simulink model "full_system_nios_id3"  (R2021b)
settings: Solver=FixedStepDiscrete  StartTime=0.0  StopTime=250000  RelTol=1e-3
model workspace (MAT data in the model file):
  out_size = 0
undefined symbols (not defined in the file): betas, bias, DiscIntNeverNeededParam, mus, scale, sigmas
libraries: hdlsllib x2
settings Model: DataTypeOverride=Off  SimulationMode=accelerator  Creator=local_adm  LastModifiedBy=local_adm
settings SolverCC: AlgebraicLoopSolver=TrustRegion
settings DataIOCC: LimitDataPoints=on  SaveOutput=off  SaveTime=off
settings OptimizationCC: BlockReduction=off  ConditionallyExecuteInputs=off  DefaultParameterBehavior=Inlined  LifeSpan=inf
settings DebuggingCC: AlgebraicLoopMsg=error  SingleTaskRateTransMsg=error  ParameterPrecisionLossMsg=none  AllowSymbolicDim=off  StrictBusMsg=ErrorOnBusTreatedAsVector  SFUnexpectedBacktrackingDiag=warning  SFNoUnconditionalDefaultTransitionDiag=warning  SFExecutionAtInitializationDiag=none  SFMachineParentedDataDiag=warning  ArithmeticOperatorsInVariantConditions=warning
settings HardwareCC: ProdBitPerPointer=32  ProdBitPerSizeT=32  ProdBitPerPtrDiffT=32  ProdLargestAtomicFloat=None  ProdIntDivRoundTo=Undefined  ProdEndianess=Unspecified  ProdWordSize=32  ProdHWDeviceType=ASIC/FPGA->ASIC/FPGA  ProdEqTarget=off
settings SFSimCC: SimUseLocalCustomCode=off  CustomCodeUndefinedFunction=UseInterfaceOnly
settings RTWCC: RTWUseLocalCustomCode=off
settings CodeAppCC: StateflowObjectComments=on
settings GRTTargetCC: TargetLangStandard=C89/C90 (ANSI)
settings ConfigComp: CovScope=ReferencedModels  CovMetricSettings=dw  CovSaveCumulativeToWorkspaceVar=on  CovSaveSingleToWorkspaceVar=on  CovExternalEMLEnable=off  CovSFcnEnable=off

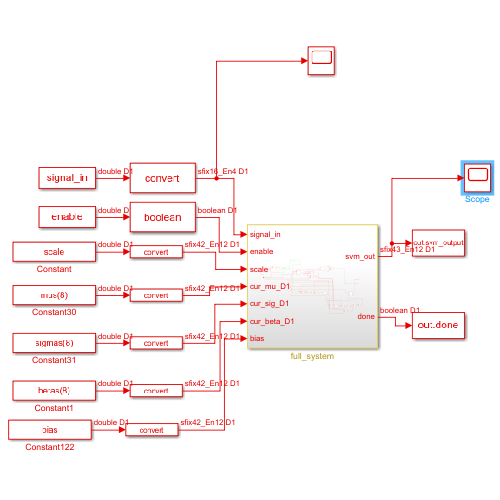
[thumbnail: Simulink's stored preview of the top-level diagram]
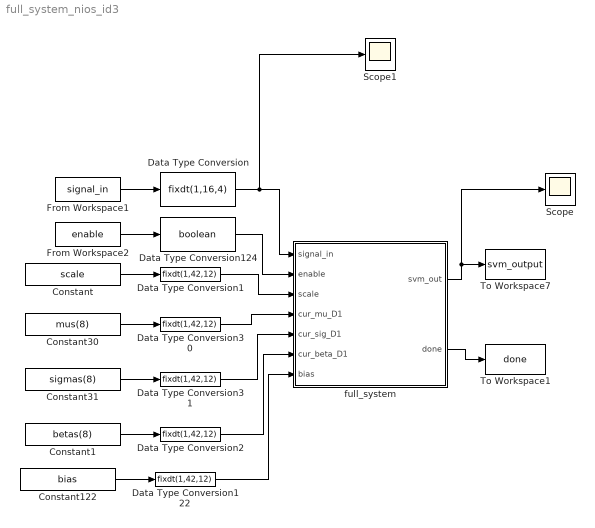
== system full_system_nios_id3 ==
  Constant : Constant  Value=scale  VectorParams1D=off  SampleTime=-1
  Constant1 : Constant  Value=betas(8)  VectorParams1D=off  SampleTime=-1
  Constant122 : Constant  Value=bias  VectorParams1D=off  SampleTime=-1
  Constant30 : Constant  Value=mus(8)  VectorParams1D=off  SampleTime=-1
  Constant31 : Constant  Value=sigmas(8)  VectorParams1D=off  SampleTime=-1
  Data Type Conversion : DataTypeConversion  OutMax=2  OutDataTypeStr=fixdt(1,16,4)
  Data Type Conversion{1..2,30..31,122} (5 alike) : DataTypeConversion  OutMax=2  OutDataTypeStr=fixdt(1,42,12)
  Data Type Conversion124 : DataTypeConversion  OutMax=1  OutDataTypeStr=boolean
  From Workspace1 : FromWorkspace  VariableName=signal_in  SampleTime=1  OutputAfterFinalValue=Setting to zero
  From Workspace2 : FromWorkspace  VariableName=enable  SampleTime=1  OutputAfterFinalValue=Setting to zero
  Scope : Scope
  Scope1 : Scope
  To Workspace1 : ToWorkspace  VariableName=done  SampleTime=-1
  To Workspace7 : ToWorkspace  VariableName=svm_output  SampleTime=-1
  full_system : Subsystem
  wires:
  full_system/2(done) -> To Workspace1/1
  From Workspace2/1 -> Data Type Conversion124/1
  Data Type Conversion30/1 -> full_system/4(cur_mu_D1)
  Data Type Conversion122/1 -> full_system/7(bias)
  Data Type Conversion31/1 -> full_system/5(cur_sig_D1)
  Data Type Conversion1/1 -> full_system/3(scale)
  Data Type Conversion124/1 -> full_system/2(enable)
  Data Type Conversion/1 -> Scope1/1, full_system/1(signal_in)
  Constant122/1 -> Data Type Conversion122/1
  full_system/1(svm_out) -> Scope/1, To Workspace7/1
  Constant30/1 -> Data Type Conversion30/1
  Constant31/1 -> Data Type Conversion31/1
  Constant/1 -> Data Type Conversion1/1
  From Workspace1/1 -> Data Type Conversion/1
  Constant1/1 -> Data Type Conversion2/1
  Data Type Conversion2/1 -> full_system/6(cur_beta_D1)

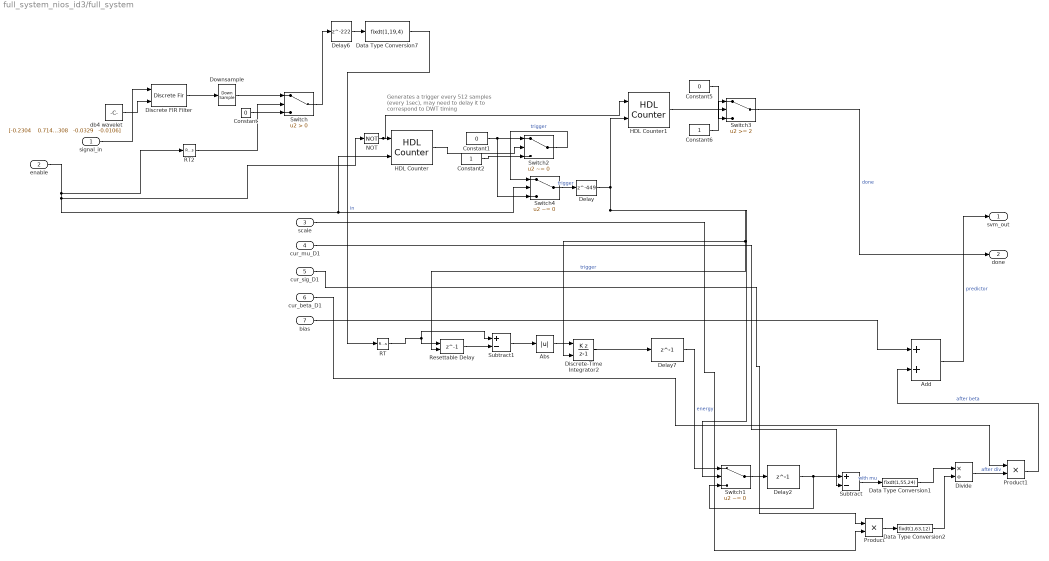
== system full_system_nios_id3/full_system ==
  note: Generates a trigger every 512 samples (every 1sec), may need to delay it to correspond to DWT timing
  signal_in : Inport
  enable : Inport  Port=2
  scale : Inport  Port=3
  cur_mu_D1 : Inport  Port=4
  cur_sig_D1 : Inport  Port=5
  cur_beta_D1 : Inport  Port=6
  bias : Inport  Port=7
  Abs : Abs
  Add : Sum
  Constant : Constant  Value=0  OutDataTypeStr=Inherit: Inherit via back propagation  SampleTime=-1
  Constant1 : Constant  Value=0  VectorParams1D=off  OutDataTypeStr=boolean  SampleTime=-1
  Constant2 : Constant  VectorParams1D=off  OutDataTypeStr=boolean  SampleTime=-1
  Constant5 : Constant  Value=0  VectorParams1D=off  OutDataTypeStr=boolean  SampleTime=-1
  Constant6 : Constant  VectorParams1D=off  OutDataTypeStr=boolean  SampleTime=-1
  Data Type Conversion1 : DataTypeConversion  OutMax=2  OutDataTypeStr=fixdt(1,55,24)
  Data Type Conversion2 : DataTypeConversion  OutMax=2  OutDataTypeStr=fixdt(1,63,12)
  Data Type Conversion7 : DataTypeConversion  OutDataTypeStr=fixdt(1,19,4)
  Delay : Delay  DelayLength=449  InitialCondition=0  UseCircularBuffer=on
  Delay2 : Delay  DelayLength=1  InitialCondition=0  UseCircularBuffer=on
  Delay6 : Delay  DelayLength=222
  Delay7 : Delay  DelayLength=1  InitialCondition=0  UseCircularBuffer=on
  Discrete FIR Filter : DiscreteFir  CoefSource=Input port
      settings: InputPortMap=u0,u1
  Discrete-Time Integrator2 : DiscreteIntegrator  IntegratorMethod=Accumulation: Backward Euler  ExternalReset=rising  SampleTime=-1  ICPrevOutput=DiscIntNeverNeededParam  ICPrevScaledInput=DiscIntNeverNeededParam
  Divide : Product  Inputs=*/  OutDataTypeStr=fixdt(1,42,12)  RndMeth=Zero  SaturateOnIntegerOverflow=on
  Downsample : DownSample  phase=1  RateOptions=Allow multirate processing
  HDL Counter : hdlsllib/Sources/HDL Counter  CountType=Count limited  CountInit=0  CountStep=1  CountMax=511  CountFromType=Initial value  CountFrom=0  CountResetPort=on  CountLoadPort=off  CountEnbPort=on  CountDirPort=off  CountHitOutputPort=off  CountDataType=Unsigned  CountWordLen=9  CountFracLen=0  CountSampTime=1
  HDL Counter1 : hdlsllib/Sources/HDL Counter  CountType=Count limited  CountInit=0  CountStep=1  CountMax=2  CountFromType=Initial value  CountFrom=0  CountResetPort=on  CountLoadPort=off  CountEnbPort=on  CountDirPort=off  CountHitOutputPort=off  CountDataType=Unsigned  CountWordLen=4  CountFracLen=0  CountSampTime=1
  NOT : Logic  Operator=NOT  IconShape=distinctive  AllPortsSameDT=off  OutDataTypeStr=boolean
  Product : Product
  Product1 : Product  OutDataTypeStr=fixdt(1,32,12)
  RT : RateTransition  OutPortSampleTime=1
  RT2 : RateTransition  OutPortSampleTime=2
  Resettable Delay : Delay  DelayLength=1  ExternalReset=Level
      settings: InputPortMap=u0,r5
  Subtract : Sum  Inputs=+-
  Subtract1 : Sum  Inputs=+-
  Switch : Switch  Criteria=u2 > Threshold
  Switch1 : Switch  Criteria=u2 ~= 0
  Switch2 : Switch  Criteria=u2 ~= 0
  Switch3 : Switch  Threshold=2
  Switch4 : Switch  Criteria=u2 ~= 0
  db4 wavelet : Constant  Value="[-0.2304    0.7148   -0.6309   -0.0280    0.1870    0.0308   -0.0329   -0.0106]"  OutDataTypeStr=Inherit: Inherit via back propagation  SampleTime=-1
  svm_out : Outport
  done : Outport  Port=2
  wires:
  Switch/1 -> Delay6/1
  Delay6/1 -> Data Type Conversion7/1
  RT2/1 -> Switch/2
  Downsample/1 -> Switch/1
  Discrete FIR Filter/1 -> Downsample/1
  Constant/1 -> Switch/3
  signal_in/1 -> Discrete FIR Filter/1
  db4 wavelet/1 -> Discrete FIR Filter/2
  Resettable Delay/1 -> Subtract1/2
  Subtract1/1 -> Abs/1
  Abs/1 -> Discrete-Time Integrator2/1
  Discrete-Time Integrator2/1 -> Delay7/1
  RT/1 -> Resettable Delay/1, Subtract1/1
  Data Type Conversion7/1 -> RT/1  "in"
  Switch3/1 -> done/1  "done"
  HDL Counter1/1 -> Switch3/2
  Constant6/1 -> Switch3/1
  Constant5/1 -> Switch3/3
  NOT/1 -> HDL Counter1/1, HDL Counter/1
  Switch4/1 -> Delay/1  "trigger"
  Switch2/1 -> Switch4/1  "trigger"
  enable/1 -> Switch4/2, HDL Counter/2, NOT/1, RT2/1
  Add/1 -> svm_out/1  "predictor"
  bias/1 -> Add/1
  Delay/1 -> Switch1/2, Resettable Delay/2, Discrete-Time Integrator2/2, HDL Counter1/2  "trigger"
  Constant1/1 -> Switch4/3, Switch2/1
  Constant2/1 -> Switch2/3
  HDL Counter/1 -> Switch2/2
  Divide/1 -> Product1/2  "after div"
  Product1/1 -> Add/2  "after beta"
  Data Type Conversion2/1 -> Divide/2
  cur_beta_D1/1 -> Product1/1
  Switch1/1 -> Delay2/1
  scale/1 -> Product/2
  Product/1 -> Data Type Conversion2/1
  Delay7/1 -> Switch1/1  "energy"
  Data Type Conversion1/1 -> Divide/1
  cur_sig_D1/1 -> Product/1
  Subtract/1 -> Data Type Conversion1/1  "with mu"
  Delay2/1 -> Subtract/1, Switch1/3
  cur_mu_D1/1 -> Subtract/2
